simulink model "part1_dynamic_model"  (R2020b)
settings: Solver=FixedStepAuto  StartTime=0.0  StopTime=200  FixedStep=0.01  RelTol=1e-3
values from neighbouring files (symbols this model uses):
  ceta = 3    [part1_test_K1.m]    (also in part2_PID_feedback.m)
  K1 = i + (300-length_iter/2)    [part1_test_K1.m]    (also in part2_PID_feedback.m = 0.1)
  K2 = 0.05    [part1_test_K1.m]    (also in part2_PID_feedback.m)
  T = 20    [part1_test_K1.m]    (also in part2_PID_feedback.m)
  tao = 5    [part1_test_K1.m]    (also in part2_PID_feedback.m)
settings Model: Creator=Weiyang  LastModifiedBy=Weiyang
settings DataIOCC: SaveFormat=Array  ReturnWorkspaceOutputs=off  LoggingToFile=on

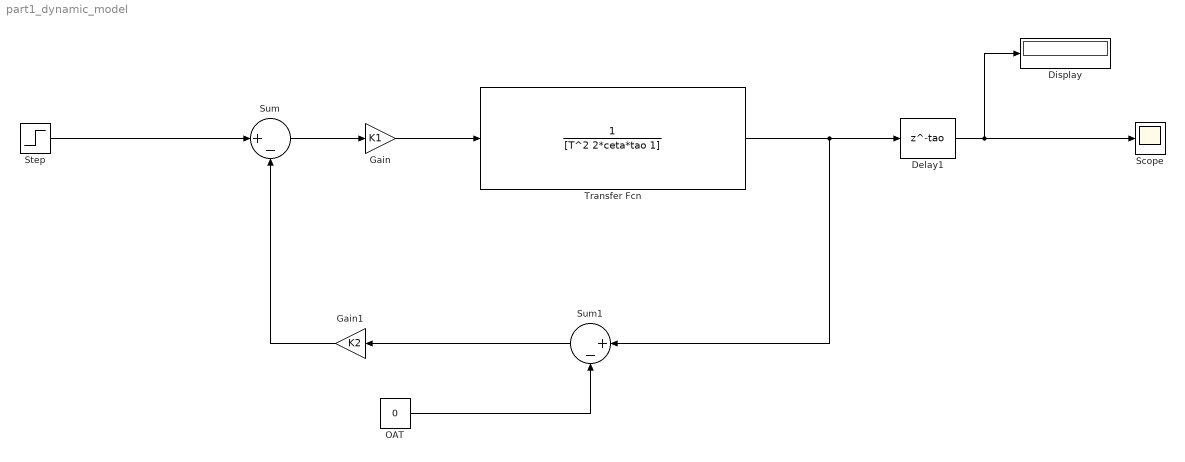
== system part1_dynamic_model ==
  Delay1 : Delay  DelayLength=tao  InputProcessing=Columns as channels (frame based)
  Display : Display
  Gain : Gain  Gain=K1
  Gain1 : Gain  Gain=K2
  OAT : Constant  Value=0
  Scope : Scope
  Step : Step  Time=0.01  SampleTime=0
  Sum : Sum  Inputs=|+-
  Sum1 : Sum  Inputs=|+-
  Transfer Fcn : TransferFcn  Denominator=[T^2 2*ceta*tao 1]
  wires:
  Sum/1 -> Gain/1
  Gain/1 -> Transfer Fcn/1
  Gain1/1 -> Sum/2
  Sum1/1 -> Gain1/1
  Transfer Fcn/1 -> Sum1/1, Delay1/1
  OAT/1 -> Sum1/2
  Delay1/1 -> Scope/1, Display/1
  Step/1 -> Sum/1
